simulink library "NEdgeDetector_lib"  (R2018b)
settings: Solver=VariableStepAuto  StartTime=0.0  StopTime=10.0  RelTol=1e-3
undefined symbols (not defined in the file or in its folder): fswParams
settings Model: Creator=Taylor  LastModifiedBy=Taylor

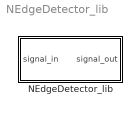
== system NEdgeDetector_lib ==
  NEdgeDetector_lib : Subsystem  mask{DelayLength=fswParams.estimation.triad_cycles, InitialCondition=fswParams.estimation.ic.activate_triad}
      mask prompts: DelayLength "Number of sample times to delay rise in output signal after a rise in input signal"; InitialCondition "Initial condition of the internal delayed state"
      mask TypeOptions DelayLength: Delay/DelayLength
      mask TypeOptions InitialCondition: Delay/InitialCondition
      mask DialogControl DescTextVar Prompt: A custom implementation of the Simulink block "Edge Detector" to enable custom delay lengths. Input signal *must* be a scalar Boolean.

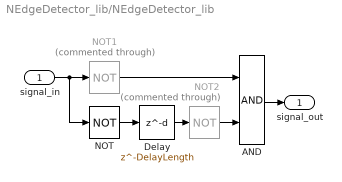
== system NEdgeDetector_lib/NEdgeDetector_lib ==
  signal_in : Inport  OutDataTypeStr=boolean  PortDimensions=1
  AND : Logic  AllPortsSameDT=off  OutDataTypeStr=boolean
  Delay : Delay  DelayLength=DelayLength  InitialCondition=InitialCondition
  NOT : Logic  Operator=NOT  AllPortsSameDT=off  OutDataTypeStr=boolean
  NOT1 : Logic  Commented=through  Operator=NOT  AllPortsSameDT=off  OutDataTypeStr=boolean
  NOT2 : Logic  Commented=through  Operator=NOT  AllPortsSameDT=off  OutDataTypeStr=boolean
  signal_out : Outport
  wires:
  Delay/1 -> NOT2/1
  NOT2/1 -> AND/2
  NOT1/1 -> AND/1
  signal_in/1 -> NOT/1, NOT1/1
  AND/1 -> signal_out/1
  NOT/1 -> Delay/1
